simulink model "bh_COMP_MODEL_Lag4dof"  (R2016b)
settings: Solver=ode15s  StartTime=0.0  StopTime=1000  FixedStep=0.001  RelTol=1e-5  EnableMultiTasking=on
undefined symbols (not defined in the file or in its folder): b1_damp, b2_damp, b3_damp, b4_damp, g, L1x, L1y, L1z, L2x, L2y, L2z, L3x, L3y, L3z, mass1, mass2, mass3, mass4, Rturn, theta1_0, theta1_dot_0, theta2_0, theta2_dot_0, theta3_0, theta3_dot_0, theta4_0, theta4_dot_0
settings Model: Creator=bhorton  LastModifiedBy=bhorton
settings SolverCC: ZeroCrossAlgorithm=Adaptive
settings OptimizationCC: LifeSpan=inf
settings DebuggingCC: SFUnexpectedBacktrackingDiag=warning  SFNoUnconditionalDefaultTransitionDiag=warning  SFExecutionAtInitializationDiag=none
settings GRTTargetCC: TargetLangStandard=C89/C90 (ANSI)
settings ConfigComp: CovMetricSettings=dw  CovHtmlReporting=on  CovSaveCumulativeToWorkspaceVar=on  CovSaveSingleToWorkspaceVar=on  CovExternalEMLEnable=off
settings SimscapeCC: SimscapeLogType=all  SimscapeLogDataHistory=10000  SelectedTab=Simscape Multibody

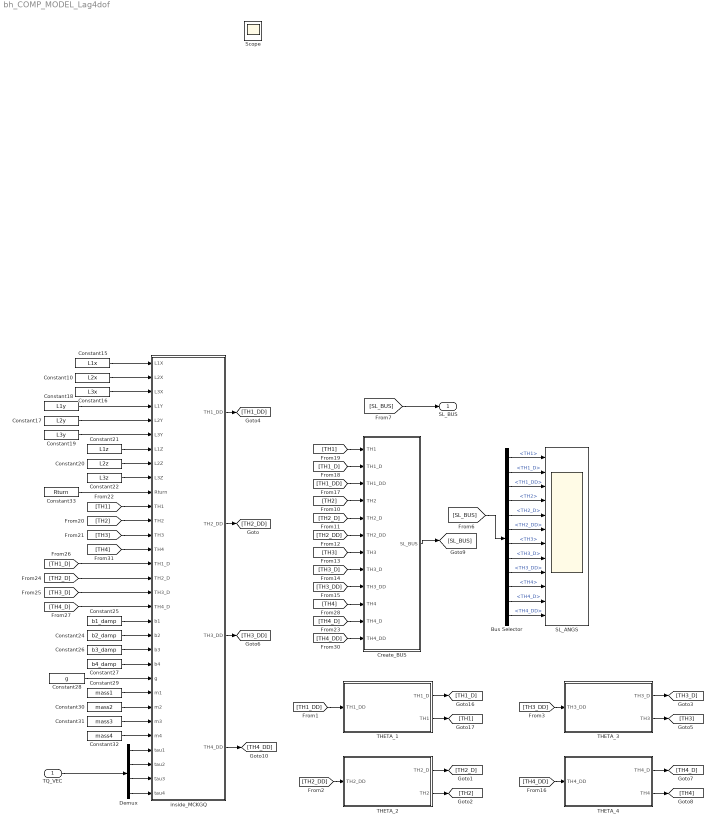
== system bh_COMP_MODEL_Lag4dof ==
  TQ_VEC : Inport
  Bus Selector : BusSelector  OutputSignals=TH1,TH1_D,TH1_DD,TH2,TH2_D,TH2_DD,TH3,TH3_D,TH3_DD,TH4,TH4_D,TH4_DD
  Constant10 : Constant  Value=L2x
  Constant15 : Constant  Value=L1x
  Constant16 : Constant  Value=L3x
  Constant17 : Constant  Value=L2y
  Constant18 : Constant  Value=L1y
  Constant19 : Constant  Value=L3y
  Constant20 : Constant  Value=L2z
  Constant21 : Constant  Value=L1z
  Constant22 : Constant  Value=L3z
  Constant24 : Constant  Value=b2_damp
  Constant25 : Constant  Value=b1_damp
  Constant26 : Constant  Value=b3_damp
  Constant27 : Constant  Value=b4_damp
  Constant28 : Constant  Value=g
  Constant29 : Constant  Value=mass1
  Constant30 : Constant  Value=mass2
  Constant31 : Constant  Value=mass3
  Constant32 : Constant  Value=mass4
  Constant33 : Constant  Value=Rturn
  Create_BUS : Subsystem
  Demux : Demux
  SL_ANGS : Scope  NumInputPorts=12
  THETA_1 : Subsystem
  THETA_2 : Subsystem
  THETA_3 : Subsystem
  THETA_4 : Subsystem
  inside_MCKGQ : Subsystem
  SL_BUS : Outport  OutDataTypeStr=Bus: BUS_DEF_4DOF
  Scope : Scope
  wires:
  [SL_BUS] -> Bus Selector/1
  [SL_BUS] -> SL_BUS/1
  Create_BUS/1(SL_BUS) -> [SL_BUS]
  Bus Selector/2 -> SL_ANGS/2  "<TH1_D>"
  Bus Selector/3 -> SL_ANGS/3  "<TH1_DD>"
  Bus Selector/1 -> SL_ANGS/1  "<TH1>"
  Bus Selector/4 -> SL_ANGS/4  "<TH2>"
  Bus Selector/5 -> SL_ANGS/5  "<TH2_D>"
  Bus Selector/6 -> SL_ANGS/6  "<TH2_DD>"
  Bus Selector/7 -> SL_ANGS/7  "<TH3>"
  Bus Selector/8 -> SL_ANGS/8  "<TH3_D>"
  Bus Selector/9 -> SL_ANGS/9  "<TH3_DD>"
  [TH2_DD] -> THETA_2/1(TH2_DD)
  THETA_2/2(TH2) -> [TH2]
  THETA_2/1(TH2_D) -> [TH2_D]
  [TH1_DD] -> THETA_1/1(TH1_DD)
  THETA_1/1(TH1_D) -> [TH1_D]
  THETA_1/2(TH1) -> [TH1]
  inside_MCKGQ/2(TH2_DD) -> [TH2_DD]
  [TH3_DD] -> THETA_3/1(TH3_DD)
  THETA_3/2(TH3) -> [TH3]
  THETA_3/1(TH3_D) -> [TH3_D]
  inside_MCKGQ/1(TH1_DD) -> [TH1_DD]
  inside_MCKGQ/3(TH3_DD) -> [TH3_DD]
  [TH3_DD] -> Create_BUS/9(TH3_DD)
  [TH1] -> Create_BUS/1(TH1)
  [TH1_D] -> Create_BUS/2(TH1_D)
  [TH1_DD] -> Create_BUS/3(TH1_DD)
  [TH2] -> Create_BUS/4(TH2)
  [TH2_D] -> Create_BUS/5(TH2_D)
  [TH2_DD] -> Create_BUS/6(TH2_DD)
  [TH3] -> Create_BUS/7(TH3)
  [TH3_D] -> Create_BUS/8(TH3_D)
  [TH4_DD] -> THETA_4/1(TH4_DD)
  THETA_4/2(TH4) -> [TH4]
  THETA_4/1(TH4_D) -> [TH4_D]
  [TH2] -> inside_MCKGQ/12(TH2)
  [TH3] -> inside_MCKGQ/13(TH3)
  [TH1] -> inside_MCKGQ/11(TH1)
  Constant10/1 -> inside_MCKGQ/2(L2X)
  Constant16/1 -> inside_MCKGQ/3(L3X)
  Constant15/1 -> inside_MCKGQ/1(L1X)
  Constant19/1 -> inside_MCKGQ/6(L3Y)
  Constant17/1 -> inside_MCKGQ/5(L2Y)
  Constant18/1 -> inside_MCKGQ/4(L1Y)
  Constant22/1 -> inside_MCKGQ/9(L3Z)
  Constant20/1 -> inside_MCKGQ/8(L2Z)
  Constant21/1 -> inside_MCKGQ/7(L1Z)
  [TH1_D] -> inside_MCKGQ/15(TH1_D)
  [TH2_D] -> inside_MCKGQ/16(TH2_D)
  [TH3_D] -> inside_MCKGQ/17(TH3_D)
  [TH4_D] -> inside_MCKGQ/18(TH4_D)
  Constant25/1 -> inside_MCKGQ/19(b1)
  Constant24/1 -> inside_MCKGQ/20(b2)
  Constant26/1 -> inside_MCKGQ/21(b3)
  Constant27/1 -> inside_MCKGQ/22(b4)
  Constant28/1 -> inside_MCKGQ/23(g)
  Constant29/1 -> inside_MCKGQ/24(m1)
  Constant30/1 -> inside_MCKGQ/25(m2)
  Constant31/1 -> inside_MCKGQ/26(m3)
  Constant32/1 -> inside_MCKGQ/27(m4)
  Constant33/1 -> inside_MCKGQ/10(Rturn)
  [TH4_D] -> Create_BUS/11(TH4_D)
  [TH4_DD] -> Create_BUS/12(TH4_DD)
  [TH4] -> Create_BUS/10(TH4)
  [TH4] -> inside_MCKGQ/14(TH4)
  inside_MCKGQ/4(TH4_DD) -> [TH4_DD]
  Bus Selector/10 -> SL_ANGS/10  "<TH4>"
  Bus Selector/11 -> SL_ANGS/11  "<TH4_D>"
  Bus Selector/12 -> SL_ANGS/12  "<TH4_DD>"
  Demux/2 -> inside_MCKGQ/29(tau2)
  Demux/3 -> inside_MCKGQ/30(tau3)
  Demux/4 -> inside_MCKGQ/31(tau4)
  TQ_VEC/1 -> Demux/1
  Demux/1 -> inside_MCKGQ/28(tau1)

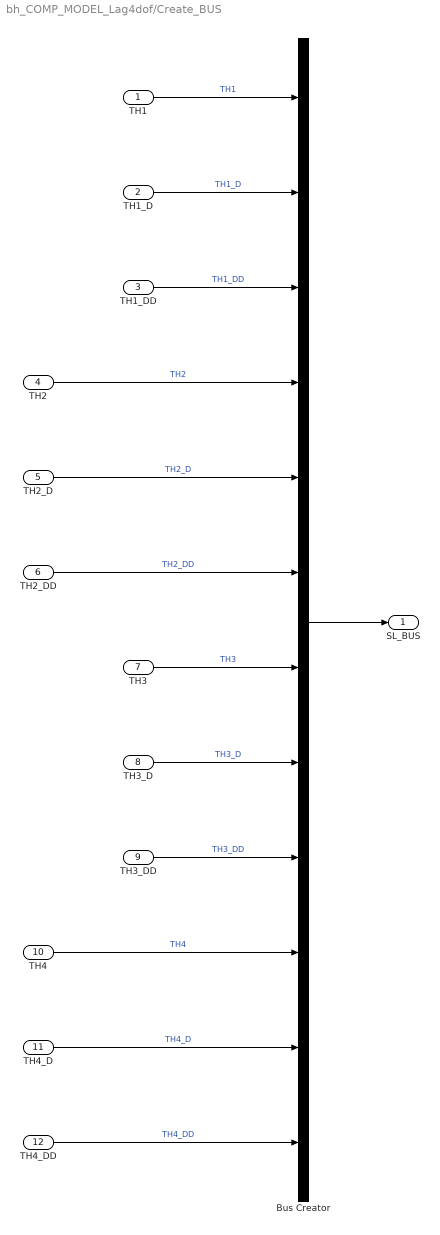
== system bh_COMP_MODEL_Lag4dof/Create_BUS ==
  TH1 : Inport
  TH1_D : Inport  Port=2
  TH1_DD : Inport  Port=3
  TH2 : Inport  Port=4
  TH2_D : Inport  Port=5
  TH2_DD : Inport  Port=6
  TH3 : Inport  Port=7
  TH3_D : Inport  Port=8
  TH3_DD : Inport  Port=9
  TH4 : Inport  Port=10
  TH4_D : Inport  Port=11
  TH4_DD : Inport  Port=12
  Bus Creator : BusCreator  Inputs=12
  SL_BUS : Outport
  wires:
  TH1_DD/1 -> Bus Creator/3  "TH1_DD"
  TH1_D/1 -> Bus Creator/2  "TH1_D"
  TH1/1 -> Bus Creator/1  "TH1"
  Bus Creator/1 -> SL_BUS/1
  TH2/1 -> Bus Creator/4  "TH2"
  TH2_D/1 -> Bus Creator/5  "TH2_D"
  TH2_DD/1 -> Bus Creator/6  "TH2_DD"
  TH3/1 -> Bus Creator/7  "TH3"
  TH3_DD/1 -> Bus Creator/9  "TH3_DD"
  TH3_D/1 -> Bus Creator/8  "TH3_D"
  TH4_DD/1 -> Bus Creator/12  "TH4_DD"
  TH4_D/1 -> Bus Creator/11  "TH4_D"
  TH4/1 -> Bus Creator/10  "TH4"

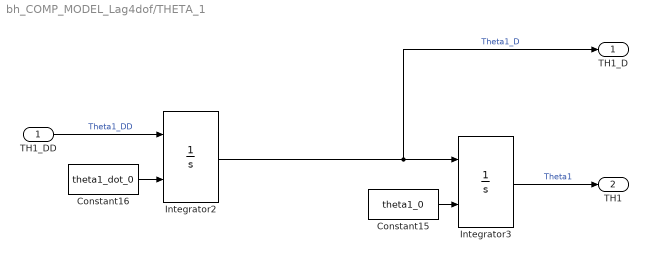
== system bh_COMP_MODEL_Lag4dof/THETA_1 ==
  TH1_DD : Inport
  Constant15 : Constant  Value=theta1_0
  Constant16 : Constant  Value=theta1_dot_0
  Integrator2 : Integrator  InitialConditionSource=external
  Integrator3 : Integrator  InitialConditionSource=external
  TH1_D : Outport
  TH1 : Outport  Port=2
  wires:
  TH1_DD/1 -> Integrator2/1  "Theta1_DD"
  Constant15/1 -> Integrator3/2
  Constant16/1 -> Integrator2/2
  Integrator3/1 -> TH1/1  "Theta1"
  Integrator2/1 -> TH1_D/1, Integrator3/1  "Theta1_D"

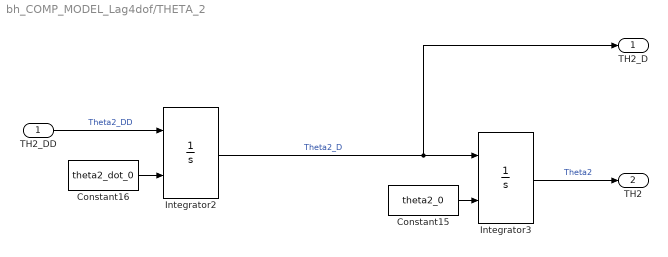
== system bh_COMP_MODEL_Lag4dof/THETA_2 ==
  TH2_DD : Inport
  Constant15 : Constant  Value=theta2_0
  Constant16 : Constant  Value=theta2_dot_0
  Integrator2 : Integrator  InitialConditionSource=external
  Integrator3 : Integrator  InitialConditionSource=external
  TH2_D : Outport
  TH2 : Outport  Port=2
  wires:
  TH2_DD/1 -> Integrator2/1  "Theta2_DD"
  Integrator2/1 -> TH2_D/1, Integrator3/1  "Theta2_D"
  Constant15/1 -> Integrator3/2
  Constant16/1 -> Integrator2/2
  Integrator3/1 -> TH2/1  "Theta2"

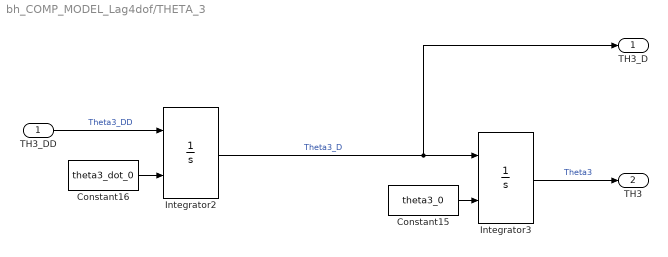
== system bh_COMP_MODEL_Lag4dof/THETA_3 ==
  TH3_DD : Inport
  Constant15 : Constant  Value=theta3_0
  Constant16 : Constant  Value=theta3_dot_0
  Integrator2 : Integrator  InitialConditionSource=external
  Integrator3 : Integrator  InitialConditionSource=external
  TH3_D : Outport
  TH3 : Outport  Port=2
  wires:
  TH3_DD/1 -> Integrator2/1  "Theta3_DD"
  Integrator2/1 -> TH3_D/1, Integrator3/1  "Theta3_D"
  Constant15/1 -> Integrator3/2
  Constant16/1 -> Integrator2/2
  Integrator3/1 -> TH3/1  "Theta3"

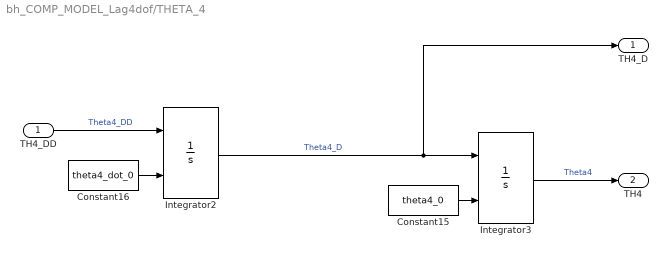
== system bh_COMP_MODEL_Lag4dof/THETA_4 ==
  TH4_DD : Inport
  Constant15 : Constant  Value=theta4_0
  Constant16 : Constant  Value=theta4_dot_0
  Integrator2 : Integrator  InitialConditionSource=external
  Integrator3 : Integrator  InitialConditionSource=external
  TH4_D : Outport
  TH4 : Outport  Port=2
  wires:
  TH4_DD/1 -> Integrator2/1  "Theta4_DD"
  Integrator2/1 -> TH4_D/1, Integrator3/1  "Theta4_D"
  Constant15/1 -> Integrator3/2
  Constant16/1 -> Integrator2/2
  Integrator3/1 -> TH4/1  "Theta4"

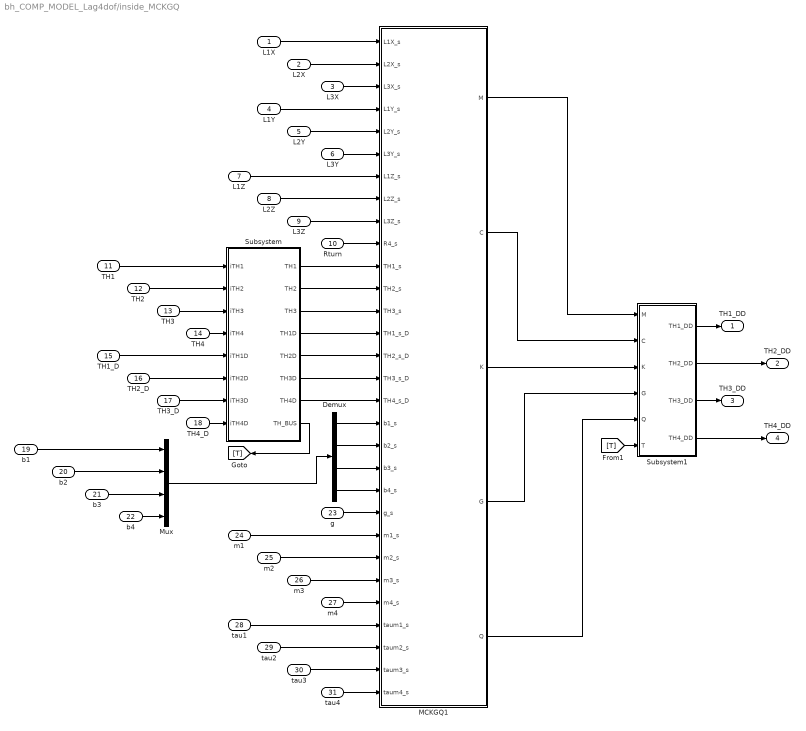
== system bh_COMP_MODEL_Lag4dof/inside_MCKGQ ==
  L1X : Inport
  L2X : Inport  Port=2
  L3X : Inport  Port=3
  L1Y : Inport  Port=4
  L2Y : Inport  Port=5
  L3Y : Inport  Port=6
  L1Z : Inport  Port=7
  L2Z : Inport  Port=8
  L3Z : Inport  Port=9
  Rturn : Inport  Port=10
  TH1 : Inport  Port=11
  TH2 : Inport  Port=12
  TH3 : Inport  Port=13
  TH4 : Inport  Port=14
  TH1_D : Inport  Port=15
  TH2_D : Inport  Port=16
  TH3_D : Inport  Port=17
  TH4_D : Inport  Port=18
  b1 : Inport  Port=19
  b2 : Inport  Port=20
  b3 : Inport  Port=21
  b4 : Inport  Port=22
  g : Inport  Port=23
  m1 : Inport  Port=24
  m2 : Inport  Port=25
  m3 : Inport  Port=26
  m4 : Inport  Port=27
  tau1 : Inport  Port=28
  tau2 : Inport  Port=29
  tau3 : Inport  Port=30
  tau4 : Inport  Port=31
  Demux : Demux
  MCKGQ1 : MATLAB Function  TreatAsAtomicUnit=on
  Mux : Mux
  Subsystem : Subsystem
  Subsystem1 : Subsystem
  TH1_DD : Outport
  TH2_DD : Outport  Port=2
  TH3_DD : Outport  Port=3
  TH4_DD : Outport  Port=4
  wires:
  m2/1 -> MCKGQ1/24(m2_s)
  m3/1 -> MCKGQ1/25(m3_s)
  m4/1 -> MCKGQ1/26(m4_s)
  tau1/1 -> MCKGQ1/27(taum1_s)
  g/1 -> MCKGQ1/22(g_s)
  m1/1 -> MCKGQ1/23(m1_s)
  TH1_D/1 -> Subsystem/5(iTH1D)
  b1/1 -> Mux/1
  b2/1 -> Mux/2
  TH3/1 -> Subsystem/3(iTH3)
  b3/1 -> Mux/3
  TH4_D/1 -> Subsystem/8(iTH4D)
  TH2_D/1 -> Subsystem/6(iTH2D)
  TH3_D/1 -> Subsystem/7(iTH3D)
  b4/1 -> Mux/4
  tau2/1 -> MCKGQ1/28(taum2_s)
  tau3/1 -> MCKGQ1/29(taum3_s)
  tau4/1 -> MCKGQ1/30(taum4_s)
  L2X/1 -> MCKGQ1/2(L2X_s)
  L3X/1 -> MCKGQ1/3(L3X_s)
  L2Y/1 -> MCKGQ1/5(L2Y_s)
  L3Y/1 -> MCKGQ1/6(L3Y_s)
  L1Y/1 -> MCKGQ1/4(L1Y_s)
  L2Z/1 -> MCKGQ1/8(L2Z_s)
  L3Z/1 -> MCKGQ1/9(L3Z_s)
  L1Z/1 -> MCKGQ1/7(L1Z_s)
  TH1/1 -> Subsystem/1(iTH1)
  Rturn/1 -> MCKGQ1/10(R4_s)
  TH2/1 -> Subsystem/2(iTH2)
  L1X/1 -> MCKGQ1/1(L1X_s)
  Subsystem/8(TH_BUS) -> [T]
  Subsystem/7(TH4D) -> MCKGQ1/17(TH4_s_D)
  Subsystem/6(TH3D) -> MCKGQ1/16(TH3_s_D)
  Subsystem/5(TH2D) -> MCKGQ1/15(TH2_s_D)
  Subsystem/4(TH1D) -> MCKGQ1/14(TH1_s_D)
  Subsystem/3(TH3) -> MCKGQ1/13(TH3_s)
  Subsystem/2(TH2) -> MCKGQ1/12(TH2_s)
  Subsystem/1(TH1) -> MCKGQ1/11(TH1_s)
  TH4/1 -> Subsystem/4(iTH4)
  Demux/1 -> MCKGQ1/18(b1_s)
  Demux/2 -> MCKGQ1/19(b2_s)
  Demux/3 -> MCKGQ1/20(b3_s)
  Demux/4 -> MCKGQ1/21(b4_s)
  Mux/1 -> Demux/1
  Subsystem1/1(TH1_DD) -> TH1_DD/1
  Subsystem1/2(TH2_DD) -> TH2_DD/1
  MCKGQ1/1(M) -> Subsystem1/1(M)
  MCKGQ1/2(C) -> Subsystem1/2(C)
  MCKGQ1/3(K) -> Subsystem1/3(K)
  MCKGQ1/4(G) -> Subsystem1/4(G)
  MCKGQ1/5(Q) -> Subsystem1/5(Q)
  [T] -> Subsystem1/6(T)
  Subsystem1/3(TH3_DD) -> TH3_DD/1
  Subsystem1/4(TH4_DD) -> TH4_DD/1

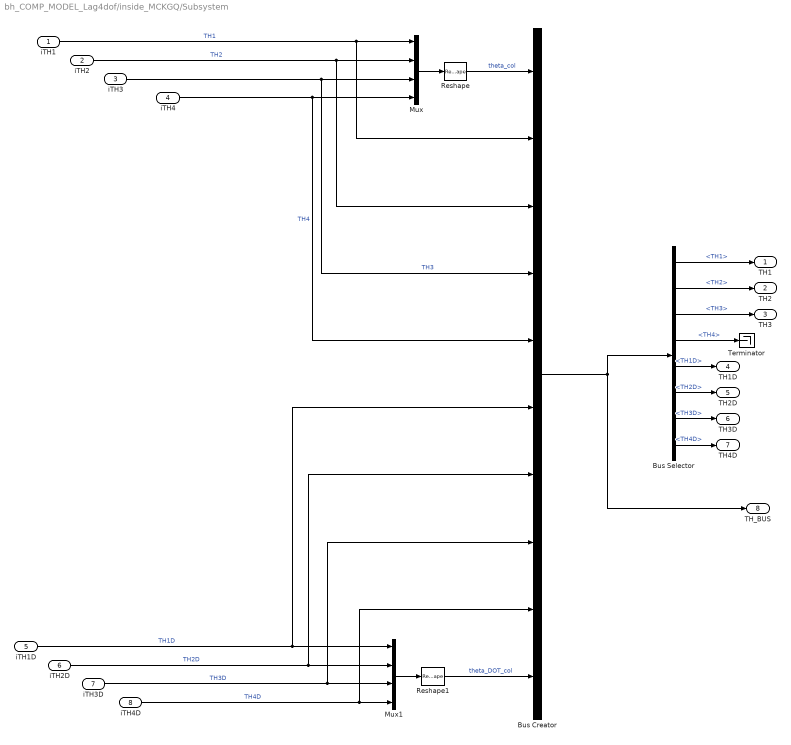
== system bh_COMP_MODEL_Lag4dof/inside_MCKGQ/Subsystem ==
  iTH1 : Inport
  iTH2 : Inport  Port=2
  iTH3 : Inport  Port=3
  iTH4 : Inport  Port=4
  iTH1D : Inport  Port=5
  iTH2D : Inport  Port=6
  iTH3D : Inport  Port=7
  iTH4D : Inport  Port=8
  Bus Creator : BusCreator  Inputs=10
  Bus Selector : BusSelector  OutputSignals=TH1,TH2,TH3,TH4,TH1D,TH2D,TH3D,TH4D
  Mux : Mux
  Mux1 : Mux
  Reshape : Reshape  OutputDimensionality=Column vector (2-D)
  Reshape1 : Reshape  OutputDimensionality=Column vector (2-D)
  Terminator : Terminator
  TH1 : Outport
  TH2 : Outport  Port=2
  TH3 : Outport  Port=3
  TH1D : Outport  Port=4
  TH2D : Outport  Port=5
  TH3D : Outport  Port=6
  TH4D : Outport  Port=7
  TH_BUS : Outport  Port=8
  wires:
  iTH2/1 -> Bus Creator/3, Mux/2  "TH2"
  iTH1/1 -> Bus Creator/2, Mux/1  "TH1"
  iTH2D/1 -> Bus Creator/7, Mux1/2  "TH2D"
  iTH1D/1 -> Bus Creator/6, Mux1/1  "TH1D"
  Mux/1 -> Reshape/1
  Mux1/1 -> Reshape1/1
  Reshape/1 -> Bus Creator/1  "theta_col"
  Reshape1/1 -> Bus Creator/10  "theta_DOT_col"
  Bus Creator/1 -> TH_BUS/1, Bus Selector/1
  iTH3D/1 -> Bus Creator/8, Mux1/3  "TH3D"
  iTH3/1 -> Bus Creator/4, Mux/3  "TH3"
  Bus Selector/1 -> TH1/1  "<TH1>"
  Bus Selector/2 -> TH2/1  "<TH2>"
  Bus Selector/3 -> TH3/1  "<TH3>"
  Bus Selector/5 -> TH1D/1  "<TH1D>"
  Bus Selector/6 -> TH2D/1  "<TH2D>"
  Bus Selector/7 -> TH3D/1  "<TH3D>"
  iTH4/1 -> Bus Creator/5, Mux/4  "TH4"
  iTH4D/1 -> Bus Creator/9, Mux1/4  "TH4D"
  Bus Selector/4 -> Terminator/1  "<TH4>"
  Bus Selector/8 -> TH4D/1  "<TH4D>"

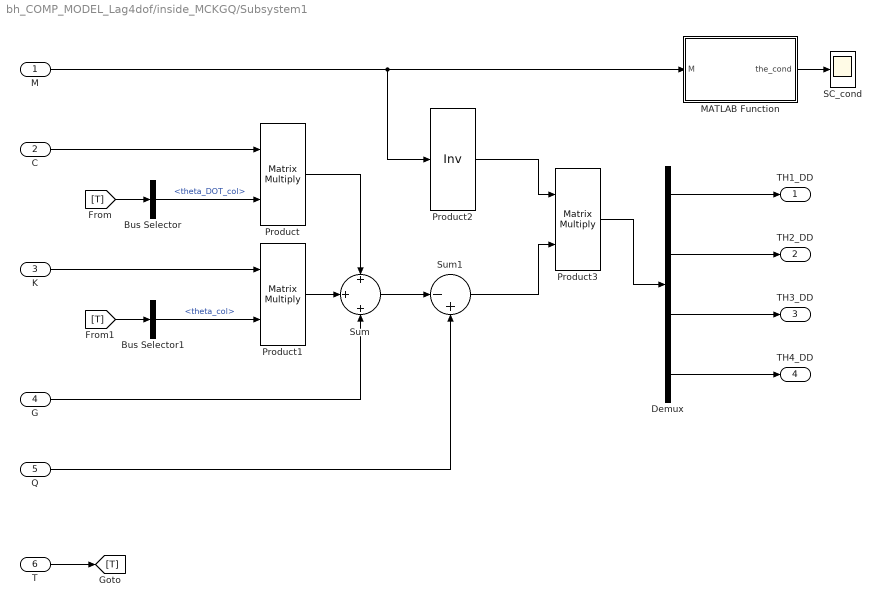
== system bh_COMP_MODEL_Lag4dof/inside_MCKGQ/Subsystem1 ==
  M : Inport
  C : Inport  Port=2
  K : Inport  Port=3
  G : Inport  Port=4
  Q : Inport  Port=5
  T : Inport  Port=6
  Bus Selector : BusSelector  OutputSignals=theta_DOT_col
  Bus Selector1 : BusSelector  OutputSignals=theta_col
  Demux : Demux
  MATLAB Function : MATLAB Function  TreatAsAtomicUnit=on
  Product : Product  Multiplication=Matrix(*)
  Product1 : Product  Multiplication=Matrix(*)
  Product2 : Product  Inputs=/  Multiplication=Matrix(*)
  Product3 : Product  Multiplication=Matrix(*)
  SC_cond : Scope
  Sum : Sum  Inputs=+|+|+
  Sum1 : Sum  Inputs=|-+
  TH1_DD : Outport
  TH2_DD : Outport  Port=2
  TH3_DD : Outport  Port=3
  TH4_DD : Outport  Port=4
  wires:
  T/1 -> [T]
  C/1 -> Product/1
  [T] -> Bus Selector/1
  Bus Selector/1 -> Product/2  "<theta_DOT_col>"
  K/1 -> Product1/1
  [T] -> Bus Selector1/1
  Bus Selector1/1 -> Product1/2  "<theta_col>"
  Q/1 -> Sum1/2
  Product1/1 -> Sum/2
  G/1 -> Sum/3
  Product/1 -> Sum/1
  Sum/1 -> Sum1/1
  M/1 -> Product2/1, MATLAB Function/1(M)
  Product2/1 -> Product3/1
  Sum1/1 -> Product3/2
  Product3/1 -> Demux/1
  Demux/1 -> TH1_DD/1
  Demux/2 -> TH2_DD/1
  MATLAB Function/1(the_cond) -> SC_cond/1
  Demux/3 -> TH3_DD/1
  Demux/4 -> TH4_DD/1

== matlab function bh_COMP_MODEL_Lag4dof/inside_MCKGQ/MCKGQ1 ==
  data: L1X_s input; M output; L2X_s input; L3X_s input; L1Y_s input; L2Y_s input; L3Y_s input; L1Z_s input; L2Z_s input; L3Z_s input; R4_s input; TH1_s input; TH2_s input; TH3_s input; TH1_s_D input; TH2_s_D input; TH3_s_D input; TH4_s_D input; b1_s input; b2_s input; b3_s input; b4_s input; g_s input; m1_s input; m2_s input; m3_s input; m4_s input; taum1_s input; taum2_s input; taum3_s input; taum4_s input; C output; K output; G output; Q output
function [M,C,K,G,Q] = MCKGQ(L1X_s,L2X_s,L3X_s,L1Y_s,L2Y_s,L3Y_s,L1Z_s,L2Z_s,L3Z_s,R4_s,TH1_s,TH2_s,TH3_s,TH1_s_D,TH2_s_D,TH3_s_D,TH4_s_D,b1_s,b2_s,b3_s,b4_s,g_s,m1_s,m2_s,m3_s,m4_s,taum1_s,taum2_s,taum3_s,taum4_s)
%#codegen

%    This function was generated by the Symbolic Math Toolbox version 7.1.
%    31-Oct-2016 17:01:09

M = reshape([L1Y_s.^2.*m1_s.*(1.0./3.0)+L1Y_s.^2.*m2_s+L1Y_s.^2.*m3_s+L2Y_s.^2.*m2_s.*(1.0./3.0)+L2Y_s.^2.*m3_s+L3Y_s.^2.*m3_s.*(1.0./3.0)+L1Z_s.^2.*m1_s.*(1.0./1.2e1)+L2Z_s.^2.*m2_s.*(1.0./1.2e1)+L3Z_s.^2.*m3_s.*(1.0./1.2e1)+L1Y_s.*L2Y_s.*m2_s.*cos(TH2_s)+L1Y_s.*L2Y_s.*m3_s.*cos(TH2_s).*2.0+L2Y_s.*L3Y_s.*m3_s.*cos(TH3_s)+L1Y_s.*L3Y_s.*m3_s.*cos(TH2_s+TH3_s),L2Y_s.^2.*m2_s.*(1.0./3.0)+L2Y_s.^2.*m3_s+L3Y_s.^2.*m3_s.*(1.0./3.0)+L2Z_s.^2.*m2_s.*(1.0./1.2e1)+L3Z_s.^2.*m3_s.*(1.0./1.2e1)+L1Y_s.*L2Y_s.*m2_s.*cos(TH2_s).*(1.0./2.0)+L1Y_s.*L2Y_s.*m3_s.*cos(TH2_s)+L2Y_s.*L3Y_s.*m3_s.*cos(TH3_s)+L1Y_s.*L3Y_s.*m3_s.*cos(TH2_s+TH3_s).*(1.0./2.0),m3_s.*(L3Y_s.^2.*4.0+L3Z_s.^2+L1Y_s.*L3Y_s.*cos(TH2_s+TH3_s).*6.0+L2Y_s.*L3Y_s.*cos(TH3_s).*6.0).*(1.0./1.2e1),0.0,L2Y_s.^2.*m2_s.*(1.0./3.0)+L2Y_s.^2.*m3_s+L3Y_s.^2.*m3_s.*(1.0./3.0)+L2Z_s.^2.*m2_s.*(1.0./1.2e1)+L3Z_s.^2.*m3_s.*(1.0./1.2e1)+L1Y_s.*L2Y_s.*m2_s.*cos(TH2_s).*(1.0./2.0)+L1Y_s.*L2Y_s.*m3_s.*cos(TH2_s)+L2Y_s.*L3Y_s.*m3_s.*cos(TH3_s)+L1Y_s.*L3Y_s.*m3_s.*cos(TH2_s+TH3_s).*(1.0./2.0),L2Y_s.^2.*m2_s.*(1.0./3.0)+L2Y_s.^2.*m3_s+L3Y_s.^2.*m3_s.*(1.0./3.0)+L2Z_s.^2.*m2_s.*(1.0./1.2e1)+L3Z_s.^2.*m3_s.*(1.0./1.2e1)+L2Y_s.*L3Y_s.*m3_s.*cos(TH3_s),m3_s.*(L3Y_s.^2.*4.0+L3Z_s.^2+L2Y_s.*L3Y_s.*cos(TH3_s).*6.0).*(1.0./1.2e1),0.0,m3_s.*(L3Y_s.^2.*4.0+L3Z_s.^2+L1Y_s.*L3Y_s.*cos(TH2_s+TH3_s).*6.0+L2Y_s.*L3Y_s.*cos(TH3_s).*6.0).*(1.0./1.2e1),m3_s.*(L3Y_s.^2.*4.0+L3Z_s.^2+L2Y_s.*L3Y_s.*cos(TH3_s).*6.0).*(1.0./1.2e1),m3_s.*(L3Y_s.^2.*4.0+L3Z_s.^2).*(1.0./1.2e1),0.0,0.0,0.0,0.0,L1X_s.^2.*m1_s.*(1.0./1.2e1)+L2X_s.^2.*m2_s.*(1.0./1.2e1)+L3X_s.^2.*m3_s.*(1.0./1.2e1)+L1Y_s.^2.*m1_s.*(1.0./6.0)+L1Y_s.^2.*m2_s.*(1.0./2.0)+L1Y_s.^2.*m3_s.*(1.0./2.0)+L2Y_s.^2.*m2_s.*(1.0./6.0)+L2Y_s.^2.*m3_s.*(1.0./2.0)+L3Y_s.^2.*m3_s.*(1.0./6.0)+L1Z_s.^2.*m1_s.*(1.0./2.4e1)+L2Z_s.^2.*m2_s.*(1.0./2.4e1)+L3Z_s.^2.*m3_s.*(1.0./2.4e1)+R4_s.^2.*m4_s.*(1.0./2.0)+L3Y_s.^2.*m3_s.*cos(TH1_s.*2.0+TH2_s.*2.0+TH3_s.*2.0).*(1.0./6.0)-L3Z_s.^2.*m3_s.*cos(TH1_s.*2.0+TH2_s.*2.0+TH3_s.*2.0).*(1.0./2.4e1)+L1Y_s.^2.*m1_s.*cos(TH1_s.*2.0).*(1.0./6.0)+L1Y_s.^2.*m2_s.*cos(TH1_s.*2.0).*(1.0./2.0)+L1Y_s.^2.*m3_s.*cos(TH1_s.*2.0).*(1.0./2.0)-L1Z_s.^2.*m1_s.*cos(TH1_s.*2.0).*(1.0./2.4e1)+L2Y_s.^2.*m2_s.*cos(TH1_s.*2.0+TH2_s.*2.0).*(1.0./6.0)+L2Y_s.^2.*m3_s.*cos(TH1_s.*2.0+TH2_s.*2.0).*(1.0./2.0)-L2Z_s.^2.*m2_s.*cos(TH1_s.*2.0+TH2_s.*2.0).*(1.0./2.4e1)+L1Y_s.*L2Y_s.*m2_s.*cos(TH2_s).*(1.0./2.0)+L1Y_s.*L2Y_s.*m3_s.*cos(TH2_s)+L2Y_s.*L3Y_s.*m3_s.*cos(TH3_s).*(1.0./2.0)+L1Y_s.*L2Y_s.*m2_s.*cos(TH1_s.*2.0+TH2_s).*(1.0./2.0)+L1Y_s.*L2Y_s.*m3_s.*cos(TH1_s.*2.0+TH2_s)+L1Y_s.*L3Y_s.*m3_s.*cos(TH1_s.*2.0+TH2_s+TH3_s).*(1.0./2.0)+L1Y_s.*L3Y_s.*m3_s.*cos(TH2_s+TH3_s).*(1.0./2.0)+L2Y_s.*L3Y_s.*m3_s.*cos(TH1_s.*2.0+TH2_s.*2.0+TH3_s).*(1.0./2.0)],[4,4]);
if nargout > 1
    C = reshape([-L1Y_s.*L3Y_s.*TH2_s_D.*m3_s.*sin(TH2_s+TH3_s)-L1Y_s.*L3Y_s.*TH3_s_D.*m3_s.*sin(TH2_s+TH3_s)-L1Y_s.*L2Y_s.*TH2_s_D.*m2_s.*sin(TH2_s)-L1Y_s.*L2Y_s.*TH2_s_D.*m3_s.*sin(TH2_s).*2.0-L2Y_s.*L3Y_s.*TH3_s_D.*m3_s.*sin(TH3_s),L1Y_s.*L3Y_s.*TH1_s_D.*m3_s.*sin(TH2_s+TH3_s).*(1.0./2.0)+L1Y_s.*L2Y_s.*TH1_s_D.*m2_s.*sin(TH2_s).*(1.0./2.0)+L1Y_s.*L2Y_s.*TH1_s_D.*m3_s.*sin(TH2_s)-L2Y_s.*L3Y_s.*TH3_s_D.*m3_s.*sin(TH3_s),L3Y_s.*m3_s.*(L1Y_s.*TH1_s_D.*sin(TH2_s+TH3_s)+L2Y_s.*TH1_s_D.*sin(TH3_s)+L2Y_s.*TH2_s_D.*sin(TH3_s).*2.0).*(1.0./2.0),TH4_s_D.*(L3Y_s.^2.*m3_s.*sin(TH1_s.*2.0+TH2_s.*2.0+TH3_s.*2.0).*4.0-L3Z_s.^2.*m3_s.*sin(TH1_s.*2.0+TH2_s.*2.0+TH3_s.*2.0)+L1Y_s.^2.*m1_s.*sin(TH1_s.*2.0).*4.0+L1Y_s.^2.*m2_s.*sin(TH1_s.*2.0).*1.2e1+L1Y_s.^2.*m3_s.*sin(TH1_s.*2.0).*1.2e1-L1Z_s.^2.*m1_s.*sin(TH1_s.*2.0)+L2Y_s.^2.*m2_s.*sin(TH1_s.*2.0+TH2_s.*2.0).*4.0+L2Y_s.^2.*m3_s.*sin(TH1_s.*2.0+TH2_s.*2.0).*1.2e1-L2Z_s.^2.*m2_s.*sin(TH1_s.*2.0+TH2_s.*2.0)+L1Y_s.*L2Y_s.*m2_s.*sin(TH1_s.*2.0+TH2_s).*1.2e1+L1Y_s.*L2Y_s.*m3_s.*sin(TH1_s.*2.0+TH2_s).*2.4e1+L1Y_s.*L3Y_s.*m3_s.*sin(TH1_s.*2.0+TH2_s+TH3_s).*1.2e1+L2Y_s.*L3Y_s.*m3_s.*sin(TH1_s.*2.0+TH2_s.*2.0+TH3_s).*1.2e1).*(-1.0./1.2e1),L1Y_s.*L3Y_s.*TH2_s_D.*m3_s.*sin(TH2_s+TH3_s).*(-1.0./2.0)-L1Y_s.*L3Y_s.*TH3_s_D.*m3_s.*sin(TH2_s+TH3_s)-L1Y_s.*L2Y_s.*TH2_s_D.*m2_s.*sin(TH2_s).*(1.0./2.0)-L1Y_s.*L2Y_s.*TH2_s_D.*m3_s.*sin(TH2_s)-L2Y_s.*L3Y_s.*TH3_s_D.*m3_s.*sin(TH3_s),-L2Y_s.*L3Y_s.*TH3_s_D.*m3_s.*sin(TH3_s),L2Y_s.*L3Y_s.*TH2_s_D.*m3_s.*sin(TH3_s).*(1.0./2.0),TH4_s_D.*(L3Y_s.^2.*m3_s.*sin(TH1_s.*2.0+TH2_s.*2.0+TH3_s.*2.0).*4.0-L3Z_s.^2.*m3_s.*sin(TH1_s.*2.0+TH2_s.*2.0+TH3_s.*2.0)+L2Y_s.^2.*m2_s.*sin(TH1_s.*2.0+TH2_s.*2.0).*4.0+L2Y_s.^2.*m3_s.*sin(TH1_s.*2.0+TH2_s.*2.0).*1.2e1-L2Z_s.^2.*m2_s.*sin(TH1_s.*2.0+TH2_s.*2.0)+L1Y_s.*L2Y_s.*m2_s.*sin(TH2_s).*6.0+L1Y_s.*L2Y_s.*m3_s.*sin(TH2_s).*1.2e1+L1Y_s.*L2Y_s.*m2_s.*sin(TH1_s.*2.0+TH2_s).*6.0+L1Y_s.*L2Y_s.*m3_s.*sin(TH1_s.*2.0+TH2_s).*1.2e1+L1Y_s.*L3Y_s.*m3_s.*sin(TH1_s.*2.0+TH2_s+TH3_s).*6.0+L1Y_s.*L3Y_s.*m3_s.*sin(TH2_s+TH3_s).*6.0+L2Y_s.*L3Y_s.*m3_s.*sin(TH1_s.*2.0+TH2_s.*2.0+TH3_s).*1.2e1).*(-1.0./1.2e1),L3Y_s.*TH3_s_D.*m3_s.*(L1Y_s.*sin(TH2_s+TH3_s)+L2Y_s.*sin(TH3_s)).*(-1.0./2.0),L2Y_s.*L3Y_s.*TH3_s_D.*m3_s.*sin(TH3_s).*(-1.0./2.0),0.0,TH4_s_D.*m3_s.*(L3Y_s.^2.*sin(TH1_s.*2.0+TH2_s.*2.0+TH3_s.*2.0).*4.0-L3Z_s.^2.*sin(TH1_s.*2.0+TH2_s.*2.0+TH3_s.*2.0)+L1Y_s.*L3Y_s.*sin(TH1_s.*2.0+TH2_s+TH3_s).*6.0+L1Y_s.*L3Y_s.*sin(TH2_s+TH3_s).*6.0+L2Y_s.*L3Y_s.*sin(TH1_s.*2.0+TH2_s.*2.0+TH3_s).*6.0+L2Y_s.*L3Y_s.*sin(TH3_s).*6.0).*(-1.0./1.2e1),TH4_s_D.*(L3Y_s.^2.*m3_s.*sin(TH1_s.*2.0+TH2_s.*2.0+TH3_s.*2.0).*4.0-L3Z_s.^2.*m3_s.*sin(TH1_s.*2.0+TH2_s.*2.0+TH3_s.*2.0)+L1Y_s.^2.*m1_s.*sin(TH1_s.*2.0).*4.0+L1Y_s.^2.*m2_s.*sin(TH1_s.*2.0).*1.2e1+L1Y_s.^2.*m3_s.*sin(TH1_s.*2.0).*1.2e1-L1Z_s.^2.*m1_s.*sin(TH1_s.*2.0)+L2Y_s.^2.*m2_s.*sin(TH1_s.*2.0+TH2_s.*2.0).*4.0+L2Y_s.^2.*m3_s.*sin(TH1_s.*2.0+TH2_s.*2.0).*1.2e1-L2Z_s.^2.*m2_s.*sin(TH1_s.*2.0+TH2_s.*2.0)+L1Y_s.*L2Y_s.*m2_s.*sin(TH1_s.*2.0+TH2_s).*1.2e1+L1Y_s.*L2Y_s.*m3_s.*sin(TH1_s.*2.0+TH2_s).*2.4e1+L1Y_s.*L3Y_s.*m3_s.*sin(TH1_s.*2.0+TH2_s+TH3_s).*1.2e1+L2Y_s.*L3Y_s.*m3_s.*sin(TH1_s.*2.0+TH2_s.*2.0+TH3_s).*1.2e1).*(1.0./2.4e1),TH4_s_D.*(L3Y_s.^2.*m3_s.*sin(TH1_s.*2.0+TH2_s.*2.0+TH3_s.*2.0).*4.0-L3Z_s.^2.*m3_s.*sin(TH1_s.*2.0+TH2_s.*2.0+TH3_s.*2.0)+L2Y_s.^2.*m2_s.*sin(TH1_s.*2.0+TH2_s.*2.0).*4.0+L2Y_s.^2.*m3_s.*sin(TH1_s.*2.0+TH2_s.*2.0).*1.2e1-L2Z_s.^2.*m2_s.*sin(TH1_s.*2.0+TH2_s.*2.0)+L1Y_s.*L2Y_s.*m2_s.*sin(TH2_s).*6.0+L1Y_s.*L2Y_s.*m3_s.*sin(TH2_s).*1.2e1+L1Y_s.*L2Y_s.*m2_s.*sin(TH1_s.*2.0+TH2_s).*6.0+L1Y_s.*L2Y_s.*m3_s.*sin(TH1_s.*2.0+TH2_s).*1.2e1+L1Y_s.*L3Y_s.*m3_s.*sin(TH1_s.*2.0+TH2_s+TH3_s).*6.0+L1Y_s.*L3Y_s.*m3_s.*sin(TH2_s+TH3_s).*6.0+L2Y_s.*L3Y_s.*m3_s.*sin(TH1_s.*2.0+TH2_s.*2.0+TH3_s).*1.2e1).*(1.0./2.4e1),TH4_s_D.*m3_s.*(L3Y_s.^2.*sin(TH1_s.*2.0+TH2_s.*2.0+TH3_s.*2.0).*4.0-L3Z_s.^2.*sin(TH1_s.*2.0+TH2_s.*2.0+TH3_s.*2.0)+L1Y_s.*L3Y_s.*sin(TH1_s.*2.0+TH2_s+TH3_s).*6.0+L1Y_s.*L3Y_s.*sin(TH2_s+TH3_s).*6.0+L2Y_s.*L3Y_s.*sin(TH1_s.*2.0+TH2_s.*2.0+TH3_s).*6.0+L2Y_s.*L3Y_s.*sin(TH3_s).*6.0).*(1.0./2.4e1),0.0],[4,4]);
end
if nargout > 2
    K = reshape([0.0,0.0,0.0,0.0,0.0,0.0,0.0,0.0,0.0,0.0,0.0,0.0,0.0,0.0,0.0,0.0],[4,4]);
end
if nargout > 3
    G = [g_s.*(L2Y_s.*m2_s.*cos(TH1_s+TH2_s)+L2Y_s.*m3_s.*cos(TH1_s+TH2_s).*2.0+L1Y_s.*m1_s.*cos(TH1_s)+L1Y_s.*m2_s.*cos(TH1_s).*2.0+L1Y_s.*m3_s.*cos(TH1_s).*2.0+L3Y_s.*m3_s.*cos(TH1_s+TH2_s+TH3_s)).*(1.0./2.0);L3Y_s.*g_s.*m3_s.*cos(TH1_s+TH2_s+TH3_s).*(1.0./2.0)+L2Y_s.*g_s.*m2_s.*cos(TH1_s+TH2_s).*(1.0./2.0)+L2Y_s.*g_s.*m3_s.*cos(TH1_s+TH2_s);L3Y_s.*g_s.*m3_s.*cos(TH1_s+TH2_s+TH3_s).*(1.0./2.0);0.0];
end
if nargout > 4
    Q = [taum1_s-TH1_s_D.*b1_s;taum2_s-TH2_s_D.*b2_s;taum3_s-TH3_s_D.*b3_s;taum4_s-TH4_s_D.*b4_s];
end

== matlab function bh_COMP_MODEL_Lag4dof/inside_MCKGQ/Subsystem1/MATLAB Function ==
  data: M input; the_cond output
function the_cond = COND(M)
%#codegen

the_cond = cond(M);

end
